simulink model "CLIK"  (R2020b)
settings: Solver=VariableStepAuto  StartTime=0.0  StopTime=T(end)+3  RelTol=1e-3
undefined symbols (not defined in the file): a1, a2, d0, DiscIntNeverNeededParam, q0
settings Model: Creator=damia  LastModifiedBy=Utente
settings DataIOCC: ReturnWorkspaceOutputs=off
settings DebuggingCC: ArithmeticOperatorsInVariantConditions=warning
settings SFSimCC: CustomCodeUndefinedFunction=UseInterfaceOnly

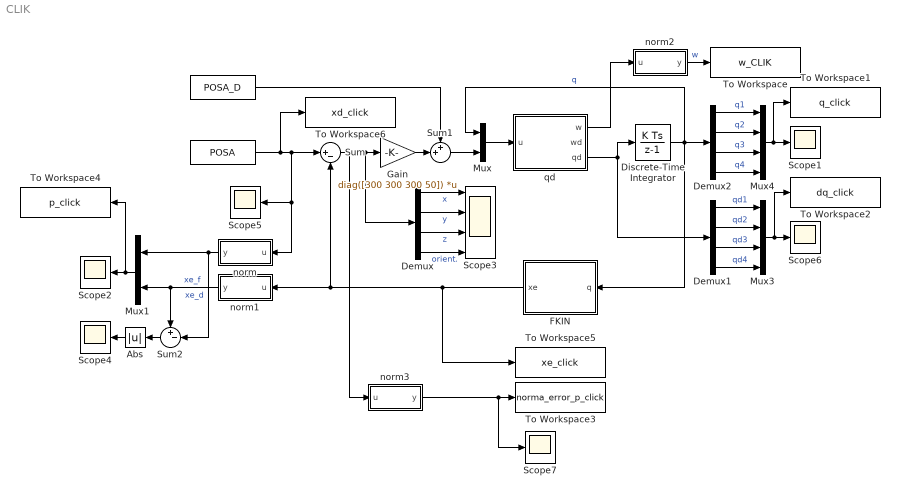
== system CLIK ==
  " " : FromWorkspace  VariableName=POSA  SampleTime=0.001
  " " : FromWorkspace  VariableName=POSA_D  SampleTime=0.001
  Abs : Abs
  Demux : Demux
  Demux1 : Demux
  Demux2 : Demux
  Discrete-Time Integrator : DiscreteIntegrator  InitialCondition=q0  SampleTime=1e-3  ICPrevOutput=DiscIntNeverNeededParam  ICPrevScaledInput=DiscIntNeverNeededParam
  FKIN : MATLAB Function  TreatAsAtomicUnit=on
  Gain : Gain  Gain=diag([300 300 300 50])  Multiplication=Matrix(K*u)
  Mux : Mux  Inputs=2
  Mux1 : Mux  Inputs=2
  Mux3 : Mux
  Mux4 : Mux
  Scope{1..2,4..7} (6 alike) : Scope
  Scope3 : Scope  NumInputPorts=4
  Sum : Sum  Inputs=|+-
  Sum1 : Sum  Inputs=++|
  Sum2 : Sum  Inputs=+-|
  To Workspace : ToWorkspace  VariableName=w_CLIK  SaveFormat=Timeseries  SampleTime=-1
  To Workspace1 : ToWorkspace  VariableName=q_click  SaveFormat=Timeseries  SampleTime=-1
  To Workspace2 : ToWorkspace  VariableName=dq_click  SaveFormat=Timeseries  SampleTime=-1
  To Workspace3 : ToWorkspace  VariableName=norma_error_p_click  SaveFormat=Timeseries  SampleTime=-1
  To Workspace4 : ToWorkspace  VariableName=p_click  SaveFormat=Timeseries  SampleTime=-1
  To Workspace5 : ToWorkspace  VariableName=xe_click  SaveFormat=Timeseries  SampleTime=-1
  To Workspace6 : ToWorkspace  VariableName=xd_click  SaveFormat=Timeseries  SampleTime=-1
  norm : MATLAB Function  TreatAsAtomicUnit=on
  norm1 : MATLAB Function  TreatAsAtomicUnit=on
  norm2 : MATLAB Function  TreatAsAtomicUnit=on
  norm3 : MATLAB Function  TreatAsAtomicUnit=on
  qd : MATLAB Function  TreatAsAtomicUnit=on
  wires:
  " "/1 -> Sum1/1
  qd/3(qd) -> Discrete-Time Integrator/1, Demux1/1
  Mux/1 -> qd/1(u)
  Gain/1 -> Sum1/2
  Sum1/1 -> Mux/2
  Discrete-Time Integrator/1 -> Demux2/1, Mux/1, FKIN/1(q)  "q"
  Sum/1 -> norm3/1(u), Demux/1, Gain/1
  Mux1/1 -> To Workspace4/1, Scope2/1
  FKIN/1(xe) -> To Workspace5/1, Sum/2, norm1/1(u)
  norm/1(y) -> Mux1/1, Sum2/2  "xe_d"
  norm1/1(y) -> Sum2/1, Mux1/2  "xe_f"
  Demux/1 -> Scope3/1  "x"
  Demux/2 -> Scope3/2  "y"
  Demux/3 -> Scope3/3  "z"
  Demux/4 -> Scope3/4  "orient."
  Demux1/3 -> Mux3/3  "qd3"
  Demux1/4 -> Mux3/4  "qd4"
  Demux1/1 -> Mux3/1  "qd1"
  Demux1/2 -> Mux3/2  "qd2"
  Mux3/1 -> To Workspace2/1, Scope6/1
  Demux2/3 -> Mux4/3  "q3"
  Demux2/4 -> Mux4/4  "q4"
  Demux2/1 -> Mux4/1  "q1"
  Demux2/2 -> Mux4/2  "q2"
  Mux4/1 -> To Workspace1/1, Scope1/1
  Sum2/1 -> Abs/1
  Abs/1 -> Scope4/1
  norm2/1(y) -> To Workspace/1  "w"
  " "/1 -> Scope5/1, norm/1(u), Sum/1, To Workspace6/1
  norm3/1(y) -> Scope7/1, To Workspace3/1
  qd/1(w) -> norm2/1(u)

== matlab function CLIK/qd ==
  data: w output; wd output; u input; qd output; a1 parameter; a2 parameter
function [w,wd, qd] = fcn(u, a1, a2)

q = u(1:4);
u2 = u(5:8);

% Jacobiano
J = [ -a1*sin(q(1))-a2*sin(q(1)+q(2))   -a2*sin(q(1)+q(2))  0   0   ;
       a1*cos(q(1))+a2*cos(q(1)+q(2))    a2*cos(q(1)+q(2))  0   0   ;
                   0                              0         1   0   ;
                   1                              1         0   1   ];
w=abs(det(J));              
wd = [0; a1*a2*cos(q(2)); 0; 0];
               
% Damped Least Squares
intervallo = 0.001;
k = 0.1;

if(abs(det(J))) < intervallo;
    J = J' * inv(J*J' + eye(4)*k^2);
    qd = J*(u2);
else
    qd = inv(J)*(u2);
end

== matlab function CLIK/FKIN ==
  data: q input; xe output; a2 parameter; a1 parameter; d0 parameter
function xe = fcn(q, a2, a1, d0)

theta1 = q(1);
theta2 = q(2);
d3 = q(3);
theta4 = q(4);

% Cinematica diretta
xe = [a1*cos(theta1)+a2*cos(theta1+theta2) ;
      a1*sin(theta1)+a2*sin(theta1+theta2) ;
      d3+d0;
      theta1+theta2+theta4; ];
end

== matlab function CLIK/norm ==
  data: u input; y output
function y = norm(u)
y = norm(u);

== matlab function CLIK/norm1 ==
  data: u input; y output
function y = norm(u)
y = norm(u);

== matlab function CLIK/norm2 ==
  data: u input; y output
function y = norm(u)
y = norm(u);

== matlab function CLIK/norm3 ==
  data: u input; y output
function y = norm(u)
y = norm(u);
